simulink model "Satellite_Dynamic"  (R2021b)
settings: Solver=VariableStepAuto  StartTime=0.0  StopTime=10.0  RelTol=1e-3
model workspace (MAT data in the model file):
  Satellite_Inertial = 1
undefined symbols (not defined in the file): AngularMomentum_From_RW, Satellite_Inertia, Torque_From_RW
libraries: aerolibutil x1
settings Model: Creator=DCLab  LastModifiedBy=DCLab

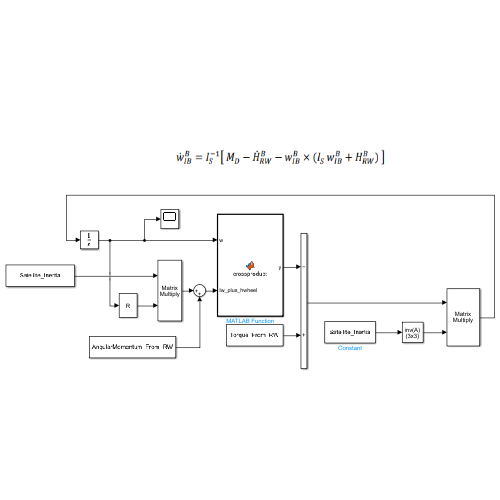
[thumbnail: Simulink's stored preview of the top-level diagram]
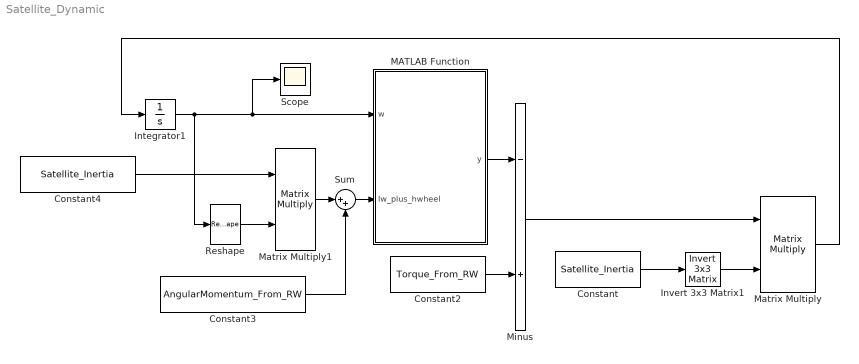
== system Satellite_Dynamic ==
  Constant : Constant  Value=Satellite_Inertia
  Constant2 : Constant  Value=Torque_From_RW
  Constant3 : Constant  Value=AngularMomentum_From_RW
  Constant4 : Constant  Value=Satellite_Inertia
  Integrator1 : Integrator
  Invert 3x3 Matrix1 : aerolibutil/Invert  3x3 Matrix
  MATLAB Function : MATLAB Function  TreatAsAtomicUnit=on
  Matrix Multiply : Product  Multiplication=Matrix(*)
  Matrix Multiply1 : Product  Multiplication=Matrix(*)
  Minus : Sum  Inputs=-+
  Reshape : Reshape  OutputDimensionality=Customize  OutputDimensions=[3,1]
  Scope : Scope
  Sum : Sum  Inputs=|++
  wires:
  MATLAB Function/1(y) -> Minus/1
  Constant2/1 -> Minus/2
  Minus/1 -> Matrix Multiply/1
  Constant/1 -> Invert 3x3 Matrix1/1
  Invert 3x3 Matrix1/1 -> Matrix Multiply/2
  Matrix Multiply/1 -> Integrator1/1
  Integrator1/1 -> Scope/1, MATLAB Function/1(w), Reshape/1
  Matrix Multiply1/1 -> Sum/1
  Constant4/1 -> Matrix Multiply1/1
  Constant3/1 -> Sum/2
  Sum/1 -> MATLAB Function/2(Iw_plus_hwheel)
  Reshape/1 -> Matrix Multiply1/2

== matlab function Satellite_Dynamic/MATLAB Function ==
  data: w input; y output; Iw_plus_hwheel input
function y = crossproduct(w,Iw_plus_hwheel)
% This block supports the Embedded MATLAB subset.
% See the help menu for details. 

%Just used to calculate the cross-product of two inputs
y = cross(w,Iw_plus_hwheel);
